simulink model "discrete_time_realistic_sim"  (R2022a)
settings: Solver=VariableStepAuto  StartTime=0.0  StopTime=5.0  RelTol=1e-3
values from neighbouring files (symbols this model uses):
  A = [0 0 0 0 0 0 40.7055790872 38.6368253303 1 0 -13.2363115295 -4.71950452077 ... (16 elements, 4x4)]    [lin_ss_model.mat]    (also in lin_state_space.m = [0 0     1      0)
  B = [0 0 23.29957643 8.30763585823]    [lin_ss_model.mat]    (also in lin_state_space.m = [0)
  C = eye(4)    [LQR_design.m]    (also in LQR_design_realistic.m = eye(4,4); lin_ss_model.mat = [1  0  0  0; 0  1  0  0]; lin_state_space.m = eye(2,4); main_LQR_realistic.m = eye(4,4))
  D = zeros(4,1)    [LQR_design.m]    (also in LQR_design_realistic.m; lin_ss_model.mat = [0 0]; lin_state_space.m = zeros(2,1); main_LQR_realistic.m)
  n = 0.0005    [LQR_design_realistic.m]
  Ts = 1/200    (= 0.005)    [LQR_design_realistic.m]    (also in live_sim.m = 1 / fs; main_LQR_realistic.m)
  Vsat = 5    [LQR_design_realistic.m]    (also in main_LQR_realistic.m)
  wc = 2*2*pi    (= 12.5663706144)    [LQR_design_realistic.m]    (also in live_sim.m; main_LQR_realistic.m = trial_LUT(trial_index).wc)
  x0 = [0,0,0,0]    [LQR_design.m]    (also in LQR_design_realistic.m; live_sim.m = x0; main_LQR_realistic.m = [0, disturbance_alpha*pi/180, 0, 0])
  xd = [30*pi/180,0,0,0]    [LQR_design.m]    (also in LQR_design_realistic.m; live_sim.m = xd; main_LQR_realistic.m = xd)
undefined symbols (not defined in the file or in its folder): K_control
libraries: simulink x3
settings Model: Creator=gaetc  LastModifiedBy=gaetc

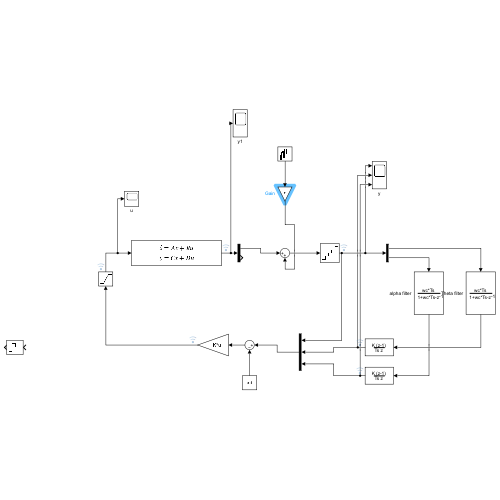
[thumbnail: Simulink's stored preview of the top-level diagram]
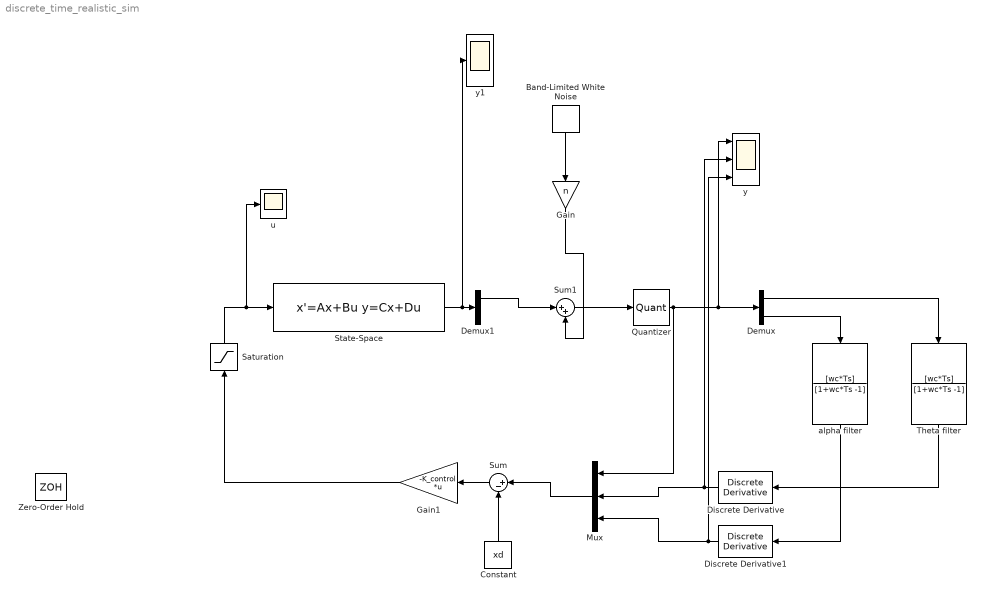
== system discrete_time_realistic_sim ==
  Band-Limited White Noise : simulink/Sources/Band-Limited White Noise  Cov=[0.1]  Ts=0.1  seed=[23341]
  Constant : Constant  Value=xd
  Demux : Demux  Outputs=2
  Demux1 : Demux  Outputs=2
  Discrete Derivative : simulink/Discrete/Discrete Derivative  gainval=1.0  ICPrevScaledInput=0.0  OutMin=[]  OutMax=[]  OutDataType=fixdt(1, 16)  OutScaling=2^-10  DoSatur=off
  Discrete Derivative1 : simulink/Discrete/Discrete Derivative  gainval=1.0  ICPrevScaledInput=0.0  OutMin=[]  OutMax=[]  OutDataType=fixdt(1, 16)  OutScaling=2^-10  DoSatur=off
  Gain : Gain  Gain=n
  Gain1 : Gain  Gain=-K_control  Multiplication=Matrix(K*u)
  Mux : Mux  Inputs=3
  Quantizer : Quantizer  QuantizationInterval=Vquant  LinearizeAsGain=off
  Saturation : Saturate  UpperLimit=Vsat  LowerLimit=-Vsat
  State-Space : StateSpace  A=A  B=B  C=C  D=D  InitialCondition=x0
  Sum : Sum  Inputs=|+-
  Sum1 : Sum  Inputs=|++
  Theta filter : DiscreteFilter  Numerator=[wc*Ts]  Denominator=[1+wc*Ts -1]
  Zero-Order Hold : ZeroOrderHold  SampleTime=Ts
  alpha filter : DiscreteFilter  Numerator=[wc*Ts]  Denominator=[1+wc*Ts -1]
  u : Scope
  y : Scope  NumInputPorts=3
  y1 : Scope
  wires:
  Demux/2 -> alpha filter/1
  Demux/1 -> Theta filter/1
  Discrete Derivative/1 -> y/2, Mux/2
  Discrete Derivative1/1 -> y/3, Mux/3
  Sum/1 -> Gain1/1
  Constant/1 -> Sum/2
  Mux/1 -> Sum/1
  Band-Limited White Noise/1 -> Gain/1
  Quantizer/1 -> Mux/1, y/1, Demux/1
  Saturation/1 -> u/1, State-Space/1
  Gain1/1 -> Saturation/1
  State-Space/1 -> y1/1, Demux1/1
  Gain/1 -> Sum1/2
  Demux1/1 -> Sum1/1
  Sum1/1 -> Quantizer/1
  alpha filter/1 -> Discrete Derivative1/1
  Theta filter/1 -> Discrete Derivative/1
